simulink library "Satellite_SlewConstrained_Controller_lib"  (R2018b)
settings: Solver=VariableStepAuto  StartTime=0.0  StopTime=10.0  RelTol=1e-3
undefined symbols (not defined in the file or in its folder): fswParams
libraries: aerolibutil x2, $bdroot x2
settings Model: Creator=colem  LastModifiedBy=colem

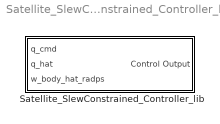
== system Satellite_SlewConstrained_Controller_lib ==
  Satellite_SlewConstrained_Controller_lib : Subsystem

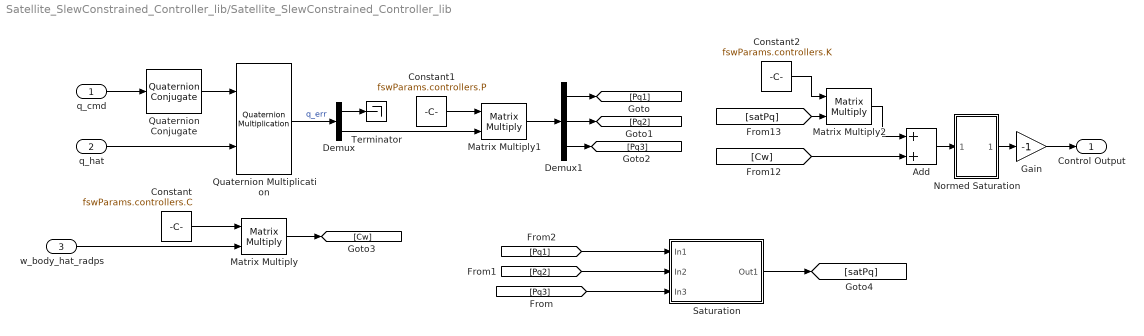
== system Satellite_SlewConstrained_Controller_lib/Satellite_SlewConstrained_Controller_lib ==
  q_cmd : Inport
  q_hat : Inport  Port=2
  w_body_hat_radps : Inport  Port=3
  Add : Sum
  Constant : Constant  Value=fswParams.controllers.C
  Constant1 : Constant  Value=fswParams.controllers.P
  Constant2 : Constant  Value=fswParams.controllers.K
  Demux : Demux  Outputs=[1 3]
  Demux1 : Demux  Outputs=3
  Gain : Gain  Gain=-1
  Matrix Multiply : Product  Multiplication=Matrix(*)
  Matrix Multiply1 : Product  Multiplication=Matrix(*)
  Matrix Multiply2 : Product  Multiplication=Matrix(*)
  Normed Saturation : Subsystem
  Quaternion Conjugate : aerolibutil/Quaternion Conjugate
      settings: SourceProductName=Aerospace Blockset  SourceProductBaseCode=AE
  Quaternion Multiplication : aerolibutil/Quaternion Multiplication
  Saturation : Subsystem
  Terminator : Terminator
  Control Output : Outport
  wires:
  Quaternion Conjugate/1 -> Quaternion Multiplication/1
  Constant1/1 -> Matrix Multiply1/1
  Demux1/3 -> [Pq3]
  Matrix Multiply1/1 -> Demux1/1
  Matrix Multiply/1 -> [Cw]
  Demux1/1 -> [Pq1]
  q_cmd/1 -> Quaternion Conjugate/1
  Constant/1 -> Matrix Multiply/1
  Demux1/2 -> [Pq2]
  w_body_hat_radps/1 -> Matrix Multiply/2
  Demux/1 -> Terminator/1
  Quaternion Multiplication/1 -> Demux/1  "q_err"
  Demux/2 -> Matrix Multiply1/2
  q_hat/1 -> Quaternion Multiplication/2
  [Pq1] -> Saturation/1(In1)
  [Pq2] -> Saturation/2(In2)
  [Pq3] -> Saturation/3(In3)
  Saturation/1(Out1) -> [satPq]
  [satPq] -> Matrix Multiply2/2
  [Cw] -> Add/2
  Normed Saturation/1(Out1) -> Gain/1
  Gain/1 -> Control Output/1
  Add/1 -> Normed Saturation/1(In1)
  Constant2/1 -> Matrix Multiply2/1
  Matrix Multiply2/1 -> Add/1

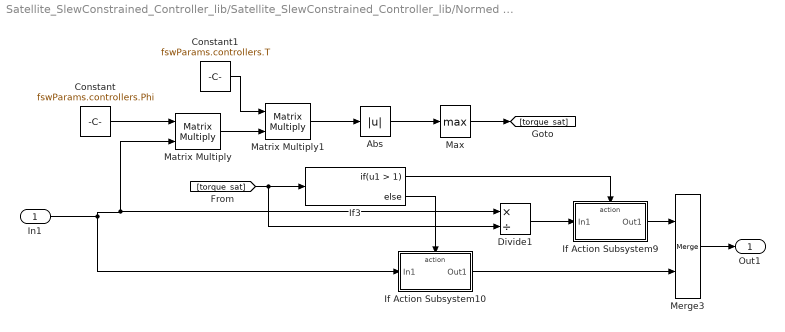
== system Satellite_SlewConstrained_Controller_lib/Satellite_SlewConstrained_Controller_lib/Normed Saturation ==
  In1 : Inport
  Abs : Abs
  Constant : Constant  Value=fswParams.controllers.Phi
  Constant1 : Constant  Value=fswParams.controllers.T
  Divide1 : Product  Inputs=*/
  If Action Subsystem10 : Subsystem  TreatAsAtomicUnit=on
  If Action Subsystem9 : Subsystem  TreatAsAtomicUnit=on
  If3 : If  IfExpression=u1 > 1
  Matrix Multiply : Product  Multiplication=Matrix(*)
  Matrix Multiply1 : Product  Multiplication=Matrix(*)
  Max : MinMax  Function=max
  Merge3 : Merge
  Out1 : Outport
  wires:
  If Action Subsystem9/1(Out1) -> Merge3/1
  If3/1 -> If Action Subsystem9/Action
  If3/2 -> If Action Subsystem10/Action
  If Action Subsystem10/1(Out1) -> Merge3/2
  Merge3/1 -> Out1/1
  Divide1/1 -> If Action Subsystem9/1(In1)
  Constant/1 -> Matrix Multiply/1
  In1/1 -> Matrix Multiply/2, Divide1/1, If Action Subsystem10/1(In1)
  Matrix Multiply/1 -> Matrix Multiply1/2
  Constant1/1 -> Matrix Multiply1/1
  Matrix Multiply1/1 -> Abs/1
  Abs/1 -> Max/1
  [torque_sat] -> Divide1/2, If3/1
  Max/1 -> [torque_sat]

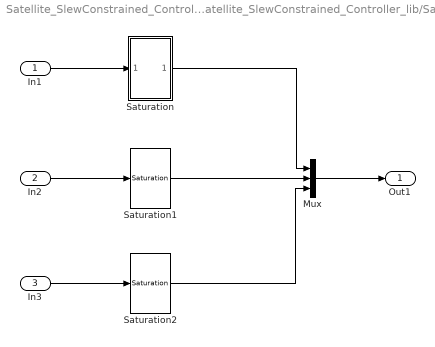
== system Satellite_SlewConstrained_Controller_lib/Satellite_SlewConstrained_Controller_lib/Saturation ==
  In1 : Inport
  In2 : Inport  Port=2
  In3 : Inport  Port=3
  Mux : Mux  Inputs=3
  Saturation : Subsystem
  Saturation1 : $bdroot/Satellite_SlewConstrained_Controller_lib/Saturation/Saturation  SystemSampleTime=-1
  Saturation2 : $bdroot/Satellite_SlewConstrained_Controller_lib/Saturation/Saturation  SystemSampleTime=-1
  Out1 : Outport
  wires:
  Mux/1 -> Out1/1
  In2/1 -> Saturation1/1
  In1/1 -> Saturation/1(In1)
  Saturation/1(Out1) -> Mux/1
  Saturation1/1 -> Mux/2
  In3/1 -> Saturation2/1
  Saturation2/1 -> Mux/3

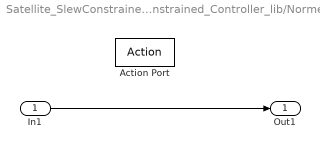
== system Satellite_SlewConstrained_Controller_lib/Satellite_SlewConstrained_Controller_lib/Normed Saturation/If Action Subsystem10 ==
  In1 : Inport
  Action Port : ActionPort  ActionType=else
  Out1 : Outport
  wires:
  In1/1 -> Out1/1

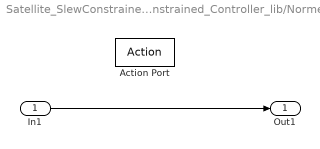
== system Satellite_SlewConstrained_Controller_lib/Satellite_SlewConstrained_Controller_lib/Normed Saturation/If Action Subsystem9 ==
  In1 : Inport
  Action Port : ActionPort  ActionType=then
  Out1 : Outport
  wires:
  In1/1 -> Out1/1

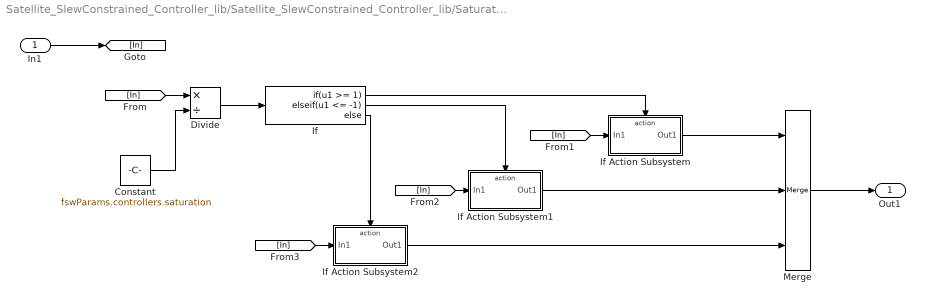
== system Satellite_SlewConstrained_Controller_lib/Satellite_SlewConstrained_Controller_lib/Saturation/Saturation ==
  In1 : Inport
  Constant : Constant  Value=fswParams.controllers.saturation
  Divide : Product  Inputs=*/
  If : If  IfExpression=u1 >= 1  ElseIfExpressions=u1 <= -1
  If Action Subsystem : Subsystem  TreatAsAtomicUnit=on
  If Action Subsystem1 : Subsystem  TreatAsAtomicUnit=on
  If Action Subsystem2 : Subsystem  TreatAsAtomicUnit=on
  Merge : Merge  Inputs=3
  Out1 : Outport
  wires:
  [In] -> If Action Subsystem/1(In1)
  If/2 -> If Action Subsystem1/Action
  If Action Subsystem2/1(Out1) -> Merge/3
  If Action Subsystem1/1(Out1) -> Merge/2
  If/1 -> If Action Subsystem/Action
  [In] -> If Action Subsystem2/1(In1)
  If Action Subsystem/1(Out1) -> Merge/1
  [In] -> If Action Subsystem1/1(In1)
  If/3 -> If Action Subsystem2/Action
  Merge/1 -> Out1/1
  In1/1 -> [In]
  [In] -> Divide/1
  Divide/1 -> If/1
  Constant/1 -> Divide/2

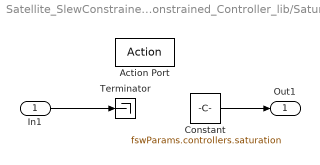
== system Satellite_SlewConstrained_Controller_lib/Satellite_SlewConstrained_Controller_lib/Saturation/Saturation/If Action Subsystem ==
  In1 : Inport
  Action Port : ActionPort  ActionType=then
  Constant : Constant  Value=fswParams.controllers.saturation
  Terminator : Terminator
  Out1 : Outport
  wires:
  In1/1 -> Terminator/1
  Constant/1 -> Out1/1

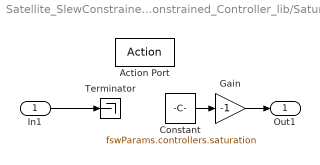
== system Satellite_SlewConstrained_Controller_lib/Satellite_SlewConstrained_Controller_lib/Saturation/Saturation/If Action Subsystem1 ==
  In1 : Inport
  Action Port : ActionPort  ActionType=elseif
  Constant : Constant  Value=fswParams.controllers.saturation
  Gain : Gain  Gain=-1
  Terminator : Terminator
  Out1 : Outport
  wires:
  In1/1 -> Terminator/1
  Constant/1 -> Gain/1
  Gain/1 -> Out1/1

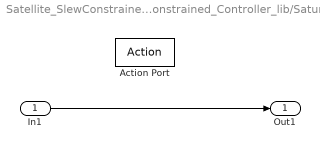
== system Satellite_SlewConstrained_Controller_lib/Satellite_SlewConstrained_Controller_lib/Saturation/Saturation/If Action Subsystem2 ==
  In1 : Inport
  Action Port : ActionPort  ActionType=else
  Out1 : Outport
  wires:
  In1/1 -> Out1/1
